simulink model "scd3busMicrogridDroopControlFidelityLevels2Inv"  (R2025b)
settings: Solver=ode15s  StartTime=0.0  StopTime=24  RelTol=1e-3
PreLoadFcn:
  | scd3busMicrogridDroopControlDataFidelityLevels2Inv;
  | 
  | %% Controller variants
  | % Create variant controls for converter controller. Controller has two
  | % different levels of fidelity: Averaged, AveragedPulse, Pulse
  | Averaged = Simulink.VariantExpression;
  | Averaged.Condition = 'fidelity==scd3busMicrogridDroopControl_variants_enum.Low';
  | Pulse = Simulink.VariantExpression;
  | Pulse.Condition = 'fidelity==scd3busMicrogridDroopControl_variants_enum.High';
  | 
  | %% Plant variants
  | % Create variant controls for converter plant. Plant has three different
  | % levels of fidelity.
  | AveragedNonSwitch = Simulink.VariantExpression;
  | AveragedNonSwitch.Condition = 'fidelity==scd3busMicrogridDroopControl_variants_enum.Low';
  | PulseSwitch = Simulink.VariantExpression;
  | PulseSwitch.Condition = 'fidelity==scd3busMicrogridDroopControl_variants_enum.High';
  | 
  | %% Set up variables ready for simulation
  | fidelity = scd3busMicrogridDroopControl_variants_enum.High;
  | Ts = 5e-6;
  | Ts_V = 1e-6;
  | Tsc = 1e-4;
  | Tsc_V = 5e-4;
values from neighbouring files (symbols this model uses):
  consensus_enable = 1    [scd3busMicrogridDroopControlDataFidelityLevels3Inv.m]
  fgrid = 60    [scd3busMicrogridDroopControlDataFidelityLevels.m]    (also in scd3busMicrogridDroopControlDataFidelityLevels3Inv.m)
  Kdroop_fp1 = 0.03/2    (= 0.015)    [scd3busMicrogridDroopControlDataFidelityLevels3Inv.m]
  Kdroop_fp2 = 0.03/2    (= 0.015)    [scd3busMicrogridDroopControlDataFidelityLevels3Inv.m]
  Kdroop_vq1 = 0.05/2    (= 0.025)    [scd3busMicrogridDroopControlDataFidelityLevels3Inv.m]
  Kdroop_vq2 = 0.05/2    (= 0.025)    [scd3busMicrogridDroopControlDataFidelityLevels3Inv.m]
  Ki_vd = 850    [scd3busMicrogridDroopControlDataFidelityLevels.m]    (also in scd3busMicrogridDroopControlDataFidelityLevels3Inv.m)
  Ki_vq = 850    [scd3busMicrogridDroopControlDataFidelityLevels.m]    (also in scd3busMicrogridDroopControlDataFidelityLevels3Inv.m)
  Kp_vd = 0.36    [scd3busMicrogridDroopControlDataFidelityLevels.m]    (also in scd3busMicrogridDroopControlDataFidelityLevels3Inv.m)
  Kp_vq = 0.36    [scd3busMicrogridDroopControlDataFidelityLevels.m]    (also in scd3busMicrogridDroopControlDataFidelityLevels3Inv.m)
  Vdc1 = 1000    [scd3busMicrogridDroopControlDataFidelityLevels.m]    (also in scd3busMicrogridDroopControlDataFidelityLevels3Inv.m)
  Vdc2 = 1000    [scd3busMicrogridDroopControlDataFidelityLevels.m]    (also in scd3busMicrogridDroopControlDataFidelityLevels3Inv.m)
  Vrms = 380    [scd3busMicrogridDroopControlDataFidelityLevels.m]    (also in scd3busMicrogridDroopControlDataFidelityLevels3Inv.m)
undefined symbols (not defined in the file or in its folder): DiscIntNeverNeededParam
libraries: ee_lib x29, nesl_utility x29, fl_lib x17, eeTransforms x4, eeSinusoidalMeasurement x4, slpidlib x4, eePwmGeneratorTwoLevel x2, eePowerMeasurement x2, simulink x2, SignalEditorBlockLib x1
(part 1 of 3)
Description:
  | Three-Phase 3 Bus Low-Inertia Microgrid Droop Control Example
settings Model: SimulationMode=rapid-accelerator  Creator=The MathWorks, Inc.  LastModifiedBy=Alex
settings SolverCC: MaxZcPerStep=1.0
settings DataIOCC: SaveOutput=off  DSMLogging=off  SaveTime=off  ReturnWorkspaceOutputs=off
settings OptimizationCC: ReuseModelBlockBuffer=off
settings DebuggingCC: StateNameClashWarn=warning
settings ModelReferenceCC: EnableRefExpFcnMdlSchedulingChecks=on
settings RTWCC: GPUComputeCapability=3.5
settings SimscapeCC: SimscapeNormalizeSystem=off

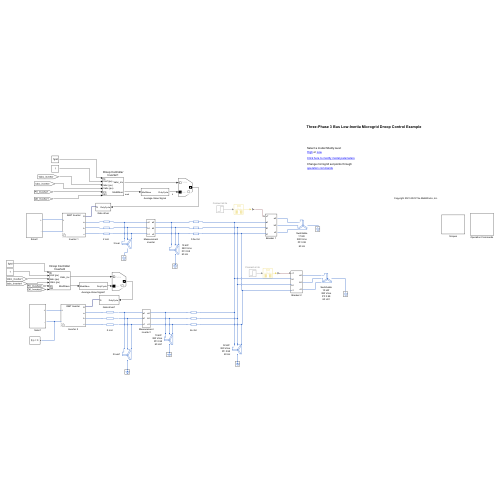
[thumbnail: Simulink's stored preview of the top-level diagram]
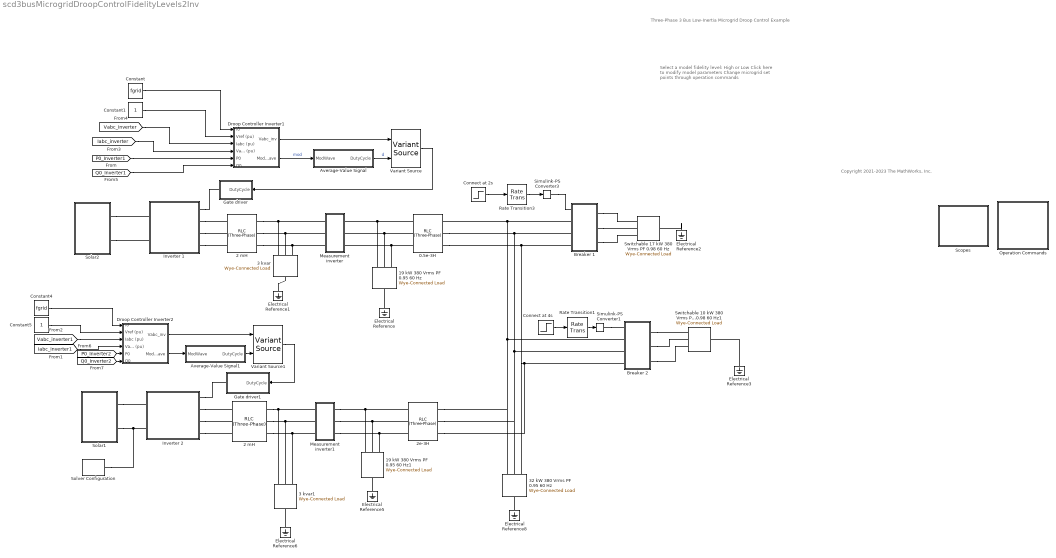
== system scd3busMicrogridDroopControlFidelityLevels2Inv ==
  note: Three-Phase 3 Bus Low-Inertia Microgrid Droop Control Example
  note: Copyright 2021-2023 The MathWorks, Inc.
  note: Select a model fidelity level:
      | High or Low
      |
      | Click here to modify model parameters
      |
      | Change microgrid set points through operation commands
  "0.5e-3H " : ee_lib/Passive/RLC Assemblies/RLC (Three-Phase)  port_option=ee.enum.threePhasePort.expanded  component_structure=ee.enum.rlc.structure.SeriesRL  R=0.02 Ohm  L=0.2e-3 H  C=1 F  R_parasitic=1e-6 Ohm  G_parasitic=1e-6 1/Ohm  IL_specify=on  IL_priority=High  IL=[0, 0, 0] A  IL_nominal_specify=off  IL_nominal_value=1  IL_nominal_unit=A  VC_specify=on  VC_priority=High  VC=[0, 0, 0] V  VC_nominal_specify=off  VC_nominal_value=1  VC_nominal_unit=V
      settings: InternalSimscapePortConfiguration="{\"Bottom\":[],\"Left\":[{\"id\":\"a1\",\"label\":\"a1\",\"type\":\"foundation.electrical.electrical\"},{\"id\":\"b1\",\"label\":\"b1\",\"type\":\"foundation.electrical.electrical\"},{\"id\":\"c1\",\"label\":\"c1\",\"type\":\"foundation.electrical.electrical\"}],\"Right\":[{\"id\":\"a2\",\"label\":\"a2\",\"type\":\"foundation.electrical.electrical\"},{\"id\":\"b2\",\"label\":\"b2\",\"type\":\"foundation.electrical.electrical\"},{\"id\":\"c2\",\"label\":\"c2\",\"type\":\"foundation.electrical.electrical\"}],\"Top\":[]}"
  19 kW 380 Vrms PF 0.95 60 Hz : ee_lib/Passive/RLC Assemblies/Wye-Connected Load  port_option=ee.enum.threePhasePort.expanded  parameterization=2  component_structure=3  component_structure_PQ=ee.enum.rlc.structure.ParallelRL  R=1 Ohm  L=0.001 H  C=1e-6 F  VRated=Vrms V  FRated=fgrid Hz  P=19000 W  Qpos=19000*sqrt(1-0.95^2)/0.95 V*A  Qneg=-3000 V*A  R_parasitic=1e-6 Ohm  G_parasitic=1e-6 1/Ohm  R_parasitic_PQ=1e-6 Ohm  G_parasitic_PQ=1e-6 1/Ohm  Vmag0=380 V  Vang0=0 deg  Freq0=60 Hz  IL_specify=on  IL_priority=High  IL=[ 0 0 0 ] A  IL_nominal_specify=off  IL_nominal_value=1  IL_nominal_unit=A  VC_specify=on  VC_priority=High  VC=[ 0 0 0 ] V  VC_nominal_specify=off  VC_nominal_value=1  VC_nominal_unit=V
      settings: InternalSimscapePortConfiguration="{\"Bottom\":[],\"Left\":[{\"id\":\"a\",\"label\":\"a\",\"type\":\"foundation.electrical.electrical\"},{\"id\":\"b\",\"label\":\"b\",\"type\":\"foundation.electrical.electrical\"},{\"id\":\"c\",\"label\":\"c\",\"type\":\"foundation.electrical.electrical\"}],\"Right\":[{\"id\":\"n\",\"label\":\"n\",\"type\":\"foundation.electrical.electrical\"}],\"Top\":[]}"
  19 kW 380 Vrms PF 0.95 60 Hz1 : ee_lib/Passive/RLC Assemblies/Wye-Connected Load  port_option=ee.enum.threePhasePort.expanded  parameterization=2  component_structure=1  component_structure_PQ=ee.enum.rlc.structure.ParallelRL  R=1 Ohm  L=0.001 H  C=1e-6 F  VRated=Vrms V  FRated=fgrid Hz  P=19000 W  Qpos=19000*sqrt(1-0.95^2)/0.95 V*A  Qneg=-3000 V*A  R_parasitic=1e-6 Ohm  G_parasitic=1e-6 1/Ohm  R_parasitic_PQ=1e-6 Ohm  G_parasitic_PQ=1e-6 1/Ohm  Vmag0=380 V  Vang0=0 deg  Freq0=60 Hz  IL_specify=on  IL_priority=High  IL=[ 0 0 0 ] A  IL_nominal_specify=off  IL_nominal_value=1  IL_nominal_unit=A  VC_specify=on  VC_priority=High  VC=[ 0 0 0 ] V  VC_nominal_specify=off  VC_nominal_value=1  VC_nominal_unit=V
      settings: InternalSimscapePortConfiguration="{\"Bottom\":[],\"Left\":[{\"id\":\"a\",\"label\":\"a\",\"type\":\"foundation.electrical.electrical\"},{\"id\":\"b\",\"label\":\"b\",\"type\":\"foundation.electrical.electrical\"},{\"id\":\"c\",\"label\":\"c\",\"type\":\"foundation.electrical.electrical\"}],\"Right\":[{\"id\":\"n\",\"label\":\"n\",\"type\":\"foundation.electrical.electrical\"}],\"Top\":[]}"
  2 mH : ee_lib/Passive/RLC Assemblies/RLC (Three-Phase)  port_option=ee.enum.threePhasePort.expanded  component_structure=ee.enum.rlc.structure.SeriesRL  R=0.02 Ohm  L=0.002 H  C=1 F  R_parasitic=1e-6 Ohm  G_parasitic=1e-6 1/Ohm  IL_specify=on  IL_priority=High  IL=[0, 0, 0] A  IL_nominal_specify=off  IL_nominal_value=1  IL_nominal_unit=A  VC_specify=on  VC_priority=High  VC=[0, 0, 0] V  VC_nominal_specify=off  VC_nominal_value=1  VC_nominal_unit=V
      settings: InternalSimscapePortConfiguration="{\"Bottom\":[],\"Left\":[{\"id\":\"a1\",\"label\":\"a1\",\"type\":\"foundation.electrical.electrical\"},{\"id\":\"b1\",\"label\":\"b1\",\"type\":\"foundation.electrical.electrical\"},{\"id\":\"c1\",\"label\":\"c1\",\"type\":\"foundation.electrical.electrical\"}],\"Right\":[{\"id\":\"a2\",\"label\":\"a2\",\"type\":\"foundation.electrical.electrical\"},{\"id\":\"b2\",\"label\":\"b2\",\"type\":\"foundation.electrical.electrical\"},{\"id\":\"c2\",\"label\":\"c2\",\"type\":\"foundation.electrical.electrical\"}],\"Top\":[]}"
  "2 mH " : ee_lib/Passive/RLC Assemblies/RLC (Three-Phase)  port_option=ee.enum.threePhasePort.expanded  component_structure=ee.enum.rlc.structure.SeriesRL  R=0.02 Ohm  L=0.002 H  C=1 F  R_parasitic=1e-6 Ohm  G_parasitic=1e-6 1/Ohm  IL_specify=on  IL_priority=High  IL=[0, 0, 0] A  IL_nominal_specify=off  IL_nominal_value=1  IL_nominal_unit=A  VC_specify=on  VC_priority=High  VC=[0, 0, 0] V  VC_nominal_specify=off  VC_nominal_value=1  VC_nominal_unit=V
      settings: InternalSimscapePortConfiguration="{\"Bottom\":[],\"Left\":[{\"id\":\"a1\",\"label\":\"a1\",\"type\":\"foundation.electrical.electrical\"},{\"id\":\"b1\",\"label\":\"b1\",\"type\":\"foundation.electrical.electrical\"},{\"id\":\"c1\",\"label\":\"c1\",\"type\":\"foundation.electrical.electrical\"}],\"Right\":[{\"id\":\"a2\",\"label\":\"a2\",\"type\":\"foundation.electrical.electrical\"},{\"id\":\"b2\",\"label\":\"b2\",\"type\":\"foundation.electrical.electrical\"},{\"id\":\"c2\",\"label\":\"c2\",\"type\":\"foundation.electrical.electrical\"}],\"Top\":[]}"
  2e-3H : ee_lib/Passive/RLC Assemblies/RLC (Three-Phase)  port_option=ee.enum.threePhasePort.expanded  component_structure=ee.enum.rlc.structure.SeriesRL  R=0.1 Ohm  L=1e-3 H  C=1 F  R_parasitic=1e-6 Ohm  G_parasitic=1e-6 1/Ohm  IL_specify=on  IL_priority=High  IL=[0, 0, 0] A  IL_nominal_specify=off  IL_nominal_value=1  IL_nominal_unit=A  VC_specify=on  VC_priority=High  VC=[0, 0, 0] V  VC_nominal_specify=off  VC_nominal_value=1  VC_nominal_unit=V
      settings: InternalSimscapePortConfiguration="{\"Bottom\":[],\"Left\":[{\"id\":\"a1\",\"label\":\"a1\",\"type\":\"foundation.electrical.electrical\"},{\"id\":\"b1\",\"label\":\"b1\",\"type\":\"foundation.electrical.electrical\"},{\"id\":\"c1\",\"label\":\"c1\",\"type\":\"foundation.electrical.electrical\"}],\"Right\":[{\"id\":\"a2\",\"label\":\"a2\",\"type\":\"foundation.electrical.electrical\"},{\"id\":\"b2\",\"label\":\"b2\",\"type\":\"foundation.electrical.electrical\"},{\"id\":\"c2\",\"label\":\"c2\",\"type\":\"foundation.electrical.electrical\"}],\"Top\":[]}"
  3 kvar : ee_lib/Passive/RLC Assemblies/Wye-Connected Load  port_option=ee.enum.threePhasePort.expanded  parameterization=2  component_structure=3  component_structure_PQ=3  R=1 Ohm  L=0.001 H  C=1e-6 F  VRated=Vrms V  FRated=fgrid Hz  P=0 W  Qpos=0 V*A  Qneg=-3000 V*A  R_parasitic=1e-6 Ohm  G_parasitic=1e-6 1/Ohm  R_parasitic_PQ=1e-6 Ohm  G_parasitic_PQ=1e-6 1/Ohm  Vmag0=380 V  Vang0=0 deg  Freq0=60 Hz  IL_specify=on  IL_priority=High  IL=[ 0 0 0 ] A  IL_nominal_specify=off  IL_nominal_value=1  IL_nominal_unit=A  VC_specify=on  VC_priority=High  VC=[ 0 0 0 ] V  VC_nominal_specify=off  VC_nominal_value=1  VC_nominal_unit=V
      settings: InternalSimscapePortConfiguration="{\"Bottom\":[],\"Left\":[{\"id\":\"a\",\"label\":\"a\",\"type\":\"foundation.electrical.electrical\"},{\"id\":\"b\",\"label\":\"b\",\"type\":\"foundation.electrical.electrical\"},{\"id\":\"c\",\"label\":\"c\",\"type\":\"foundation.electrical.electrical\"}],\"Right\":[{\"id\":\"n\",\"label\":\"n\",\"type\":\"foundation.electrical.electrical\"}],\"Top\":[]}"
  3 kvar1 : ee_lib/Passive/RLC Assemblies/Wye-Connected Load  port_option=ee.enum.threePhasePort.expanded  parameterization=ee.enum.rlc.parameterization.ratedpower  component_structure=ee.enum.rlc.structure.C  component_structure_PQ=ee.enum.rlc.structure.C  R=1 Ohm  L=0.001 H  C=1e-6 F  VRated=Vrms V  FRated=fgrid Hz  P=0 W  Qpos=0 A*V  Qneg=-3000 A*V  R_parasitic=1e-6 Ohm  G_parasitic=1e-6 1/Ohm  R_parasitic_PQ=1e-6 Ohm  G_parasitic_PQ=1e-6 1/Ohm  Vmag0=380 V  Vang0=0 deg  Freq0=60 Hz  IL_specify=on  IL_priority=High  IL=[ 0 0 0 ] A  IL_nominal_specify=off  IL_nominal_value=1  IL_nominal_unit=A  VC_specify=on  VC_priority=High  VC=[ 0 0 0 ] V  VC_nominal_specify=off  VC_nominal_value=1  VC_nominal_unit=V
      settings: InternalSimscapePortConfiguration="{\"Bottom\":[],\"Left\":[{\"id\":\"a\",\"label\":\"a\",\"type\":\"foundation.electrical.electrical\"},{\"id\":\"b\",\"label\":\"b\",\"type\":\"foundation.electrical.electrical\"},{\"id\":\"c\",\"label\":\"c\",\"type\":\"foundation.electrical.electrical\"}],\"Right\":[{\"id\":\"n\",\"label\":\"n\",\"type\":\"foundation.electrical.electrical\"}],\"Top\":[]}"
  32 kW 380 Vrms PF 0.95 60 Hz : ee_lib/Passive/RLC Assemblies/Wye-Connected Load  port_option=ee.enum.threePhasePort.expanded  parameterization=2  component_structure=3  component_structure_PQ=ee.enum.rlc.structure.ParallelRL  R=1 Ohm  L=0.001 H  C=1e-6 F  VRated=Vrms V  FRated=fgrid Hz  P=32000 W  Qpos=32000*sqrt(1-0.95^2)/0.95 V*A  Qneg=-3000 V*A  R_parasitic=1e-6 Ohm  G_parasitic=1e-6 1/Ohm  R_parasitic_PQ=1e-6 Ohm  G_parasitic_PQ=1e-6 1/Ohm  Vmag0=380 V  Vang0=0 deg  Freq0=60 Hz  IL_specify=on  IL_priority=High  IL=[ 0 0 0 ] A  IL_nominal_specify=off  IL_nominal_value=1  IL_nominal_unit=A  VC_specify=on  VC_priority=High  VC=[ 0 0 0 ] V  VC_nominal_specify=off  VC_nominal_value=1  VC_nominal_unit=V
      settings: InternalSimscapePortConfiguration="{\"Bottom\":[],\"Left\":[{\"id\":\"a\",\"label\":\"a\",\"type\":\"foundation.electrical.electrical\"},{\"id\":\"b\",\"label\":\"b\",\"type\":\"foundation.electrical.electrical\"},{\"id\":\"c\",\"label\":\"c\",\"type\":\"foundation.electrical.electrical\"}],\"Right\":[{\"id\":\"n\",\"label\":\"n\",\"type\":\"foundation.electrical.electrical\"}],\"Top\":[]}"
  Average-Value Signal : Subsystem
  Average-Value Signal1 : Subsystem
  Breaker 1 : Subsystem
  Breaker 2 : Subsystem
  Connect at 2s : Step  Time=6  SampleTime=0
  Connect at 4s : Step  Time=10  SampleTime=0
  Constant : Constant  Value=fgrid
  Constant1 : Constant
  Constant4 : Constant  Value=fgrid
  Constant5 : Constant
  Droop Controller Inverter1 : Subsystem
  Droop Controller Inverter2 : Subsystem
  Electrical Reference{,1..3,5..6,8} (7 alike) : fl_lib/Electrical/Electrical Elements/Electrical Reference
  Gate driver : Subsystem
  Gate driver1 : Subsystem
  Inverter 1 : Subsystem  Variant=on  VariantControl=Choice
  Inverter 2 : Subsystem  Variant=on  VariantControl=Choice
  Measurement inverter : Subsystem
  Measurement inverter1 : Subsystem
  Operation Commands : Subsystem
  Rate Transition1 : RateTransition  Integrity=off  OutPortSampleTimeOpt=Inherit
  Rate Transition3 : RateTransition  Integrity=off  OutPortSampleTimeOpt=Inherit
  Scopes : Subsystem
  Simulink-PS Converter1 : nesl_utility/Simulink-PS Converter  PhysicalDomain=network_engine_domain  SubClassName=ps_input  LeftPortType=input  RightPortType=output  PseudoPeriodic=off  Frequencies=[]  NoiseDistribution=none  NoiseParameters=[]  Unit=1  AffineConversion=off  FilteringAndDerivatives=provide  SimscapeFilterOrder=1  InputFilterTimeConstant=0.001  UdotUserProvided=0
  Simulink-PS Converter3 : nesl_utility/Simulink-PS Converter  PhysicalDomain=network_engine_domain  SubClassName=ps_input  LeftPortType=input  RightPortType=output  PseudoPeriodic=off  Frequencies=[]  NoiseDistribution=none  NoiseParameters=[]  Unit=1  AffineConversion=off  FilteringAndDerivatives=provide  SimscapeFilterOrder=1  InputFilterTimeConstant=0.001  UdotUserProvided=0
  Solar1 : Subsystem
  Solar2 : Subsystem
  Solver Configuration : nesl_utility/Solver Configuration  PhysicalDomain=network_engine_domain  SubClassName=solver  LeftPortType=input  RightPortType=generic  Tones=[]  Harmonics=[]  SimulateNoise=off  Profile=off  UseLocalSampling=off  EnableSwitchedLinearOptims=on  FrequencyDomain=off  UseCCode=off  RelTol=0.001  AbsTol=1e-06  MinStep=1e-09  ToWorkspace=off  RevertToSquareIcSolve=off  NumHomotopyIterations=100  PhasorMode=off  PhasorModeNumHarmonics=1  ConsistencySolver=NEWTON_FTOL  IndexReductionMethod=DerivativeReplacement  DoDC=off  ResidualTolerance=1e-09  ConsistencyTolSource=GLOBAL  ConsistencyAbsTol=0.001  ConsistencyRelTol=0.001  ConsistencyTolFactor=0.001  UseLocalSolver=on  LocalSolverChoice=NE_BACKWARD_EULER_ADVANCER  ResolveIndetEquations=on  FunctionEvalNumThread=1  LocalSolverSampleTime=Ts  DoFixedCost=off  MaxNonlinIter=3  MaxModeIter=2  ComputeImpulses=off  ImpulseIterations=1  LinearAlgebra=auto  LinearAlgebraNumThread=0  EquationFormulation=NE_TIME_EF  DelaysMemoryBudget=1024  AutomaticFiltering=on  FilteringTimeConstant=0.001  PartitionStorageMethod=AS_NEEDED  PartitionMemoryBudget=1024  PartitionMethod=FAST  MultibodyUseLocalSolver=off  MultibodyLocalSolverChoice=ODE1  MultibodyLocalSolverSampleTime=0.001
  Switchable 10 kW 380 Vrms PF 0.98 60 Hz1 : ee_lib/Passive/RLC Assemblies/Wye-Connected Load  port_option=ee.enum.threePhasePort.expanded  parameterization=2  component_structure=3  component_structure_PQ=ee.enum.rlc.structure.ParallelRL  R=1 Ohm  L=0.001 H  C=1e-6 F  VRated=Vrms V  FRated=fgrid Hz  P=10000 W  Qpos=10000*sqrt(1-0.98^2)/0.98 V*A  Qneg=-3000 V*A  R_parasitic=1e-6 Ohm  G_parasitic=1e-6 1/Ohm  R_parasitic_PQ=1e-6 Ohm  G_parasitic_PQ=1e-6 1/Ohm  Vmag0=380 V  Vang0=0 deg  Freq0=60 Hz  IL_specify=on  IL_priority=High  IL=[ 0 0 0 ] A  IL_nominal_specify=off  IL_nominal_value=1  IL_nominal_unit=A  VC_specify=on  VC_priority=High  VC=[ 0 0 0 ] V  VC_nominal_specify=off  VC_nominal_value=1  VC_nominal_unit=V
      settings: InternalSimscapePortConfiguration="{\"Bottom\":[],\"Left\":[{\"id\":\"a\",\"label\":\"a\",\"type\":\"foundation.electrical.electrical\"},{\"id\":\"b\",\"label\":\"b\",\"type\":\"foundation.electrical.electrical\"},{\"id\":\"c\",\"label\":\"c\",\"type\":\"foundation.electrical.electrical\"}],\"Right\":[{\"id\":\"n\",\"label\":\"n\",\"type\":\"foundation.electrical.electrical\"}],\"Top\":[]}"
  Switchable 17 kW 380 Vrms PF 0.98 60 Hz : ee_lib/Passive/RLC Assemblies/Wye-Connected Load  port_option=ee.enum.threePhasePort.expanded  parameterization=2  component_structure=3  component_structure_PQ=ee.enum.rlc.structure.ParallelRL  R=1 Ohm  L=0.001 H  C=1e-6 F  VRated=Vrms V  FRated=fgrid Hz  P=17000 W  Qpos=17000*sqrt(1-0.98^2)/0.98 V*A  Qneg=-3000 V*A  R_parasitic=1e-6 Ohm  G_parasitic=1e-6 1/Ohm  R_parasitic_PQ=1e-6 Ohm  G_parasitic_PQ=1e-6 1/Ohm  Vmag0=380 V  Vang0=0 deg  Freq0=60 Hz  IL_specify=on  IL_priority=High  IL=[ 0 0 0 ] A  IL_nominal_specify=off  IL_nominal_value=1  IL_nominal_unit=A  VC_specify=on  VC_priority=High  VC=[ 0 0 0 ] V  VC_nominal_specify=off  VC_nominal_value=1  VC_nominal_unit=V
      settings: InternalSimscapePortConfiguration="{\"Bottom\":[],\"Left\":[{\"id\":\"a\",\"label\":\"a\",\"type\":\"foundation.electrical.electrical\"},{\"id\":\"b\",\"label\":\"b\",\"type\":\"foundation.electrical.electrical\"},{\"id\":\"c\",\"label\":\"c\",\"type\":\"foundation.electrical.electrical\"}],\"Right\":[{\"id\":\"n\",\"label\":\"n\",\"type\":\"foundation.electrical.electrical\"}],\"Top\":[]}"
  Variant Source : VariantSource  ShowConditionOnBlock=on  VariantControls={Pulse, Averaged}
  Variant Source1 : VariantSource  ShowConditionOnBlock=on  VariantControls={Pulse, Averaged}
  wires:
  [Vabc_inverter] -> Droop Controller Inverter1/3(Iabc (pu))
  Constant1/1 -> Droop Controller Inverter1/2(Vref (pu))
  [Iabc_inverter] -> Droop Controller Inverter1/4(Vabc (pu))
  [P0_Inverter1] -> Droop Controller Inverter1/5(P0)
  Variant Source/1 -> Gate driver/1(DutyCycle)
  Average-Value Signal/1(DutyCycle) -> Variant Source/2  "d"
  Droop Controller Inverter1/1(Vabc_inv) -> Variant Source/1
  Constant/1 -> Droop Controller Inverter1/1(f0)
  [Q0_Inverter1] -> Droop Controller Inverter1/6(Q0)
  Rate Transition3/1 -> Simulink-PS Converter3/1
  Droop Controller Inverter1/2(ModWave) -> Average-Value Signal/1(ModWave)  "mod"
  Connect at 2s/1 -> Rate Transition3/1
  Connect at 4s/1 -> Rate Transition1/1
  Rate Transition1/1 -> Simulink-PS Converter1/1
  Droop Controller Inverter2/2(ModWave) -> Average-Value Signal1/1(ModWave)
  [Q0_Inverter2] -> Droop Controller Inverter2/6(Q0)
  [P0_Inverter2] -> Droop Controller Inverter2/5(P0)
  Constant4/1 -> Droop Controller Inverter2/1(f0)
  Constant5/1 -> Droop Controller Inverter2/2(Vref (pu))
  [Iabc_inverter1] -> Droop Controller Inverter2/4(Vabc (pu))
  [Vabc_inverter1] -> Droop Controller Inverter2/3(Iabc (pu))
  Average-Value Signal1/1(DutyCycle) -> Variant Source1/2
  Droop Controller Inverter2/1(Vabc_inv) -> Variant Source1/1
  Variant Source1/1 -> Gate driver1/1(DutyCycle)
  connections:
  Measurement inverter/LConn1 -- "2 mH "/RConn1 -- 3 kvar/LConn1
  Breaker 1/LConn4 -- "0.5e-3H "/RConn3 -- Breaker 2/LConn4 -- 2e-3H/RConn3 -- 32 kW 380 Vrms PF 0.95 60 Hz/LConn3
  Measurement inverter/LConn3 -- "2 mH "/RConn3 -- 3 kvar/LConn3
  Measurement inverter/LConn2 -- "2 mH "/RConn2 -- 3 kvar/LConn2
  Electrical Reference1/LConn1 -- 3 kvar/RConn1
  Electrical Reference2/LConn1 -- Switchable 17 kW 380 Vrms PF 0.98 60 Hz/RConn1
  Breaker 1/RConn2 -- Switchable 17 kW 380 Vrms PF 0.98 60 Hz/LConn2
  Electrical Reference/LConn1 -- 19 kW 380 Vrms PF 0.95 60 Hz/RConn1
  Electrical Reference8/LConn1 -- 32 kW 380 Vrms PF 0.95 60 Hz/RConn1
  Inverter 1/LConn1 -- Gate driver/RConn1
  Inverter 1/LConn2 -- "2 mH "/LConn1
  Simulink-PS Converter3/RConn1 -- Breaker 1/LConn1
  Inverter 1/LConn4 -- "2 mH "/LConn3
  Inverter 1/LConn3 -- "2 mH "/LConn2
  Breaker 1/RConn3 -- Switchable 17 kW 380 Vrms PF 0.98 60 Hz/LConn3
  Breaker 1/RConn1 -- Switchable 17 kW 380 Vrms PF 0.98 60 Hz/LConn1
  Solar2/RConn2 -- Inverter 1/RConn2
  Solar2/RConn1 -- Inverter 1/RConn1
  Breaker 2/RConn2 -- Switchable 10 kW 380 Vrms PF 0.98 60 Hz1/LConn2
  Electrical Reference3/LConn1 -- Switchable 10 kW 380 Vrms PF 0.98 60 Hz1/RConn1
  Breaker 2/RConn3 -- Switchable 10 kW 380 Vrms PF 0.98 60 Hz1/LConn3
  Breaker 2/RConn1 -- Switchable 10 kW 380 Vrms PF 0.98 60 Hz1/LConn1
  Simulink-PS Converter1/RConn1 -- Breaker 2/LConn1
  19 kW 380 Vrms PF 0.95 60 Hz/LConn1 -- "0.5e-3H "/LConn1 -- Measurement inverter/RConn1
  19 kW 380 Vrms PF 0.95 60 Hz/LConn2 -- "0.5e-3H "/LConn2 -- Measurement inverter/RConn2
  19 kW 380 Vrms PF 0.95 60 Hz/LConn3 -- "0.5e-3H "/LConn3 -- Measurement inverter/RConn3
  Breaker 2/LConn2 -- 2e-3H/RConn1 -- 32 kW 380 Vrms PF 0.95 60 Hz/LConn1 -- Breaker 1/LConn2 -- "0.5e-3H "/RConn1
  Breaker 1/LConn3 -- "0.5e-3H "/RConn2 -- 2e-3H/RConn2 -- 32 kW 380 Vrms PF 0.95 60 Hz/LConn2 -- Breaker 2/LConn3
  Inverter 2/LConn3 -- 2 mH/LConn2
  Inverter 2/LConn4 -- 2 mH/LConn3
  Measurement inverter1/RConn1 -- 2e-3H/LConn1 -- 19 kW 380 Vrms PF 0.95 60 Hz1/LConn1
  Inverter 2/LConn2 -- 2 mH/LConn1
  Electrical Reference5/LConn1 -- 19 kW 380 Vrms PF 0.95 60 Hz1/RConn1
  2 mH/RConn1 -- Measurement inverter1/LConn1 -- 3 kvar1/LConn1
  Measurement inverter1/RConn2 -- 2e-3H/LConn2 -- 19 kW 380 Vrms PF 0.95 60 Hz1/LConn2
  Solar1/RConn1 -- Inverter 2/RConn1
  2 mH/RConn3 -- Measurement inverter1/LConn3 -- 3 kvar1/LConn3
  2e-3H/LConn3 -- Measurement inverter1/RConn3 -- 19 kW 380 Vrms PF 0.95 60 Hz1/LConn3
  Inverter 2/LConn1 -- Gate driver1/RConn1
  2 mH/RConn2 -- Measurement inverter1/LConn2 -- 3 kvar1/LConn2
  Electrical Reference6/LConn1 -- 3 kvar1/RConn1
  Solar1/RConn2 -- Solver Configuration/RConn1 -- Inverter 2/RConn2

== system scd3busMicrogridDroopControlFidelityLevels2Inv/Average-Value Signal ==
  ModWave : Inport
  Bias : Bias  Bias=1  SaturateOnIntegerOverflow=off
  Bias1 : Bias  Bias=1  SaturateOnIntegerOverflow=off
  Gain : Gain  Gain=-1
  Mod. Index1 : Gain  Gain=0.5
  Mux : Mux  Inputs=2
  Rate Transition : RateTransition  OutPortSampleTime=Ts_V
  Selector4 : Selector  InputPortWidth=6  IndexOptions=Index vector (dialog)  Indices=[1 4 2 5 3 6]  OutputSizes=1
  DutyCycle : Outport
  wires:
  Mux/1 -> Selector4/1
  Bias1/1 -> Mux/2
  Selector4/1 -> DutyCycle/1
  Rate Transition/1 -> Bias/1
  Bias/1 -> Mod. Index1/1
  Mod. Index1/1 -> Mux/1, Gain/1
  Gain/1 -> Bias1/1
  ModWave/1 -> Rate Transition/1

== system scd3busMicrogridDroopControlFidelityLevels2Inv/Average-Value Signal1 ==
  ModWave : Inport
  Bias : Bias  Bias=1  SaturateOnIntegerOverflow=off
  Bias1 : Bias  Bias=1  SaturateOnIntegerOverflow=off
  Gain : Gain  Gain=-1
  Mod. Index1 : Gain  Gain=0.5
  Mux : Mux  Inputs=2
  Rate Transition : RateTransition  OutPortSampleTime=Ts_V
  Selector4 : Selector  InputPortWidth=6  IndexOptions=Index vector (dialog)  Indices=[1 4 2 5 3 6]  OutputSizes=1
  DutyCycle : Outport
  wires:
  ModWave/1 -> Rate Transition/1
  Gain/1 -> Bias1/1
  Mod. Index1/1 -> Gain/1, Mux/1
  Bias/1 -> Mod. Index1/1
  Rate Transition/1 -> Bias/1
  Selector4/1 -> DutyCycle/1
  Bias1/1 -> Mux/2
  Mux/1 -> Selector4/1

== system scd3busMicrogridDroopControlFidelityLevels2Inv/Breaker 1 ==
  SPST Switch : ee_lib/Switches & Breakers/SPST Switch  R_closed=0.01 Ohm  G_open=1e-6 S  Threshold=0.5 V  Width=0 V  model_dynamics=0  t_on=1e-3 s  t_off=1e-3 s  initial_vT=0 V
      settings: InternalSimscapePortConfiguration="{\"Bottom\":[],\"Left\":[{\"id\":\"vT\",\"label\":\"vT\",\"type\":\"input\"},{\"id\":\"p\",\"label\":\"\",\"type\":\"foundation.electrical.electrical\"}],\"Right\":[{\"id\":\"n\",\"label\":\"\",\"type\":\"foundation.electrical.electrical\"}],\"Top\":[]}"
  SPST Switch1 : ee_lib/Switches & Breakers/SPST Switch  R_closed=0.01 Ohm  G_open=1e-6 S  Threshold=0.5 V  Width=0 V  model_dynamics=0  t_on=1e-3 s  t_off=1e-3 s  initial_vT=0 V
      settings: InternalSimscapePortConfiguration="{\"Bottom\":[],\"Left\":[{\"id\":\"vT\",\"label\":\"vT\",\"type\":\"input\"},{\"id\":\"p\",\"label\":\"\",\"type\":\"foundation.electrical.electrical\"}],\"Right\":[{\"id\":\"n\",\"label\":\"\",\"type\":\"foundation.electrical.electrical\"}],\"Top\":[]}"
  SPST Switch2 : ee_lib/Switches & Breakers/SPST Switch  R_closed=0.01 Ohm  G_open=1e-6 S  Threshold=0.5 V  Width=0 V  model_dynamics=0  t_on=1e-3 s  t_off=1e-3 s  initial_vT=0 V
      settings: InternalSimscapePortConfiguration="{\"Bottom\":[],\"Left\":[{\"id\":\"vT\",\"label\":\"vT\",\"type\":\"input\"},{\"id\":\"p\",\"label\":\"\",\"type\":\"foundation.electrical.electrical\"}],\"Right\":[{\"id\":\"n\",\"label\":\"\",\"type\":\"foundation.electrical.electrical\"}],\"Top\":[]}"
  vT : PMIOPort  Side=Left
  a1 : PMIOPort  Port=2  Side=Left
  b1 : PMIOPort  Port=3  Side=Left
  c1 : PMIOPort  Port=4  Side=Left
  a2 : PMIOPort  Port=5  Side=Right
  b2 : PMIOPort  Port=6  Side=Right
  c2 : PMIOPort  Port=7  Side=Right
  connections:
  SPST Switch1/RConn1 -- b2/RConn1
  SPST Switch2/RConn1 -- a2/RConn1
  SPST Switch/LConn1 -- SPST Switch1/LConn1 -- vT/RConn1 -- SPST Switch2/LConn1
  SPST Switch/RConn1 -- c2/RConn1
  SPST Switch2/LConn2 -- a1/RConn1
  SPST Switch/LConn2 -- c1/RConn1
  SPST Switch1/LConn2 -- b1/RConn1

== system scd3busMicrogridDroopControlFidelityLevels2Inv/Breaker 2 ==
  SPST Switch : ee_lib/Switches & Breakers/SPST Switch  R_closed=0.01 Ohm  G_open=1e-6 S  Threshold=0.5 V  Width=0 V  model_dynamics=0  t_on=1e-3 s  t_off=1e-3 s  initial_vT=0 V
      settings: InternalSimscapePortConfiguration="{\"Bottom\":[],\"Left\":[{\"id\":\"vT\",\"label\":\"vT\",\"type\":\"input\"},{\"id\":\"p\",\"label\":\"\",\"type\":\"foundation.electrical.electrical\"}],\"Right\":[{\"id\":\"n\",\"label\":\"\",\"type\":\"foundation.electrical.electrical\"}],\"Top\":[]}"
  SPST Switch1 : ee_lib/Switches & Breakers/SPST Switch  R_closed=0.01 Ohm  G_open=1e-6 S  Threshold=0.5 V  Width=0 V  model_dynamics=0  t_on=1e-3 s  t_off=1e-3 s  initial_vT=0 V
      settings: InternalSimscapePortConfiguration="{\"Bottom\":[],\"Left\":[{\"id\":\"vT\",\"label\":\"vT\",\"type\":\"input\"},{\"id\":\"p\",\"label\":\"\",\"type\":\"foundation.electrical.electrical\"}],\"Right\":[{\"id\":\"n\",\"label\":\"\",\"type\":\"foundation.electrical.electrical\"}],\"Top\":[]}"
  SPST Switch2 : ee_lib/Switches & Breakers/SPST Switch  R_closed=0.01 Ohm  G_open=1e-6 S  Threshold=0.5 V  Width=0 V  model_dynamics=0  t_on=1e-3 s  t_off=1e-3 s  initial_vT=0 V
      settings: InternalSimscapePortConfiguration="{\"Bottom\":[],\"Left\":[{\"id\":\"vT\",\"label\":\"vT\",\"type\":\"input\"},{\"id\":\"p\",\"label\":\"\",\"type\":\"foundation.electrical.electrical\"}],\"Right\":[{\"id\":\"n\",\"label\":\"\",\"type\":\"foundation.electrical.electrical\"}],\"Top\":[]}"
  vT : PMIOPort  Side=Left
  a1 : PMIOPort  Port=2  Side=Left
  b1 : PMIOPort  Port=3  Side=Left
  c1 : PMIOPort  Port=4  Side=Left
  a2 : PMIOPort  Port=5  Side=Right
  b2 : PMIOPort  Port=6  Side=Right
  c2 : PMIOPort  Port=7  Side=Right
  connections:
  SPST Switch1/RConn1 -- b2/RConn1
  SPST Switch2/RConn1 -- a2/RConn1
  SPST Switch/LConn1 -- SPST Switch1/LConn1 -- vT/RConn1 -- SPST Switch2/LConn1
  SPST Switch/RConn1 -- c2/RConn1
  SPST Switch2/LConn2 -- a1/RConn1
  SPST Switch/LConn2 -- c1/RConn1
  SPST Switch1/LConn2 -- b1/RConn1

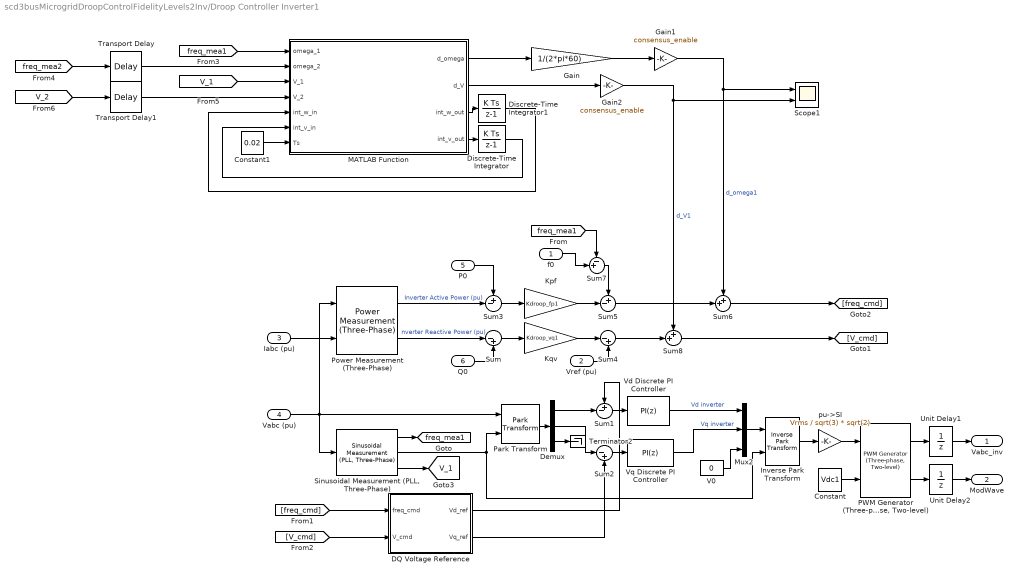
== system scd3busMicrogridDroopControlFidelityLevels2Inv/Droop Controller Inverter1 ==
  f0 : Inport
  Vref (pu) : Inport  Port=2
  Iabc (pu) : Inport  Port=3
  Vabc (pu) : Inport  Port=4
  P0 : Inport  Port=5
  Q0 : Inport  Port=6
  Constant : Constant  Value=Vdc1
  Constant1 : Constant  Value=0.02
  DQ Voltage Reference : Subsystem
  Demux : Demux  Outputs=3
  Discrete-Time Integrator : DiscreteIntegrator  SampleTime=0.02  ICPrevOutput=DiscIntNeverNeededParam  ICPrevScaledInput=DiscIntNeverNeededParam
  Discrete-Time Integrator1 : DiscreteIntegrator  SampleTime=0.02  ICPrevOutput=DiscIntNeverNeededParam  ICPrevScaledInput=DiscIntNeverNeededParam
  Gain : Gain  Gain=1/(2*pi*60)
  Gain1 : Gain  Gain=consensus_enable
  Gain2 : Gain  Gain=consensus_enable
  Inverse Park Transform : eeTransforms/Inverse Park Transform  AxisAlignment=Q-axis  PowerInvariant=off
  Kpf : Gain  Gain=Kdroop_fp1
  Kqv : Gain  Gain=Kdroop_vq1
  MATLAB Function : MATLAB Function  TreatAsAtomicUnit=on
  Mux2 : Mux  Inputs=3
  "PWM Generator (Three-phase, Two-level)" : eePwmGeneratorTwoLevel/PWM Generator (Three-phase, Two-level)  PWMMode=Continuous PWM (CPWM)  CPWMMode=SPWM: sinusoidal PWM  DPWMMode=60 DPWM: 60 degree discontinuous PWM  fsw=fsw_V  Ts=Ts_V
  Park Transform : eeTransforms/Park Transform  AxisAlignment=Q-axis  PowerInvariant=off
  Power Measurement (Three-Phase) : eePowerMeasurement/Power Measurement (Three-Phase)  LabelModeActiveChoice=Discrete  F=fgrid  K=1  Seq=Positive  Ts=Ts
  Scope1 : Scope  NumInputPorts=2
      settings: ActiveDisplayYMinimum=-0.0066314559621623061  ActiveDisplayYMaximum=0.0066314559621623061  DataLoggingVariableName=ScopeData3
  "Sinusoidal Measurement (PLL, Three-Phase)" : eeSinusoidalMeasurement/Sinusoidal Measurement (PLL, Three-Phase)  Kp_LF=180  Ki_LF=3200  F0=fgrid  Theta0=0  Ts=Ts_V
  Sum : Sum  Inputs=|-+
  Sum1 : Sum  Inputs=+-|  InputSameDT=on  SaturateOnIntegerOverflow=on  OutDataTypeStr=Inherit: Same as first input
  Sum2 : Sum  Inputs=|-+  InputSameDT=on  SaturateOnIntegerOverflow=on  OutDataTypeStr=Inherit: Same as first input
  Sum3 : Sum  Inputs=+-|
  Sum4 : Sum  Inputs=|-+
  Sum5 : Sum  Inputs=+-|
  Sum6 : Sum  Inputs=++|
  Sum7 : Sum  Inputs=-+|
  Sum8 : Sum  Inputs=++|
  Terminator2 : Terminator
  Transport Delay : TransportDelay  DelayTime=0.1
  Transport Delay1 : TransportDelay  DelayTime=0.1
  Unit Delay1 : UnitDelay  SampleTime=Ts_V  HasFrameUpgradeWarning=on
  Unit Delay2 : UnitDelay  SampleTime=Ts_V  HasFrameUpgradeWarning=on
  V0 : Constant  Value=0
  Vd Discrete PI Controller : slpidlib/PID Controller  Controller=PI  Form=Parallel  TimeDomain=Discrete-time  UseExternalTs=off  SampleTime=Ts_V  IntegratorMethod=Forward Euler  FilterMethod=Forward Euler  ControllerParametersSource=internal  P=Kp_vd  I=Ki_vd  UseKiTs=off  D=0  UseExternalDerivativeSource=off  N=100  UseFilter=on  TunerSelectOption=Transfer Function Based (PID Tuner App)  InitialConditionSource=internal  InitialConditionForIntegrator=0.62  InitialConditionForFilter=0  DifferentiatorICPrevScaledInput=0  ExternalReset=none  TrackingMode=off  Kt=1  LimitOutput=on  SatLimitsSource=internal  UpperSaturationLimit=1  LowerSaturationLimit=0  LinearizeAsGain=on  AntiWindupMode=none  Kb=1  LimitIntegrator=off  UpperIntegratorSaturationLimit=inf  LowerIntegratorSaturationLimit=-inf  POutMin=[]  POutMax=[]  IOutMin=[]  IOutMax=[]  DOutMin=[]  DOutMax=[]  NOutMin=[]  NOutMax=[]  SumOutMin=[]  SumOutMax=[]  SaturationOutMin=[]  SaturationOutMax=[]  PParamMin=[]  PParamMax=[]  IParamMin=[]  IParamMax=[]  DParamMin=[]  DParamMax=[]  NParamMin=[]  NParamMax=[]  KbParamMin=[]  KbParamMax=[]  KtParamMin=[]  KtParamMax=[]  KbOutMin=[]  KbOutMax=[]  KtOutMin=[]  KtOutMax=[]  IntegratorOutMin=[]  IntegratorOutMax=[]  FilterOutMin=[]  FilterOutMax=[]  SumI1OutMin=[]  SumI1OutMax=[]  SumI2OutMin=[]  SumI2OutMax=[]  SumI3OutMin=[]  SumI3OutMax=[]  SumI4OutMin=[]  SumI4OutMax=[]  SumDOutMin=[]  SumDOutMax=[]  DifferentiatorOutMin=[]  DifferentiatorOutMax=[]  FilterDiffOutCoefMin=[]  FilterDiffOutCoefMax=[]  ReciprocalOutMin=[]  ReciprocalOutMax=[]  SumDenOutMin=[]  SumDenOutMax=[]  SumNumOutMin=[]  SumNumOutMax=[]  DivideOutMin=[]  DivideOutMax=[]  UdiffTsProdOutMin=[]  UdiffTsProdOutMax=[]  NTsProdOutMin=[]  NTsProdOutMax=[]  UintegralTsProdOutMin=[]  UintegralTsProdOutMax=[]  UngainTsProdOutMin=[]  UngainTsProdOutMax=[]  ClampingZeroOutDataTypeStr=Inherit: Inherit via back propagation  ClampingZeroOutMin=[]  ClampingZeroOutMax=[]  FilterDenConstantOutDataTypeStr=Inherit: Inherit via back propagation  FilterDenConstantOutMin=[]  FilterDenConstantOutMax=[]  PCopyOutDataTypeStr=Inherit: Inherit via back propagation  PCopyOutMin=[]  PCopyOutMax=[]  NCopyOutDataTypeStr=Inherit: Inherit via back propagation  NCopyOutMin=[]  NCopyOutMax=[]  IntegratorContinuousStateAttributes=''  IntegratorStateMustResolveToSignalObject=off  IntegratorRTWStateStorageClass=Auto  FilterContinuousStateAttributes=''  FilterStateMustResolveToSignalObject=off  FilterRTWStateStorageClass=Auto  ParallelPVariant=InternalParameters  IdealPVariant=Disabled  IVariant=InternalParameters  DVariant=Disabled  IntegratorVariant=Discrete  SatVariant=Enabled  AWVariant=Passthrough  PCopyVariant=Disabled  TRVariant=Disabled  FdbkBlocksVariant=Forward  IdealPFdbkVariant=Disabled  SatFdbkVariant=Disabled  DerivativeFilterVariant=Disabled  NVariant=Disabled  NCopyVariant=Disabled_SignalSpec  FilterICVariant=Disabled  IntegratorICVariant=InternalICs  ExternalResetVariant=Disabled  TRSumVariant=Passthrough  SumFdbkVariant=Disabled  SumVariant=Sum_PI  TsampFilterVariant=InternalTs  TsampNgainVariant=Passthrough  TsampIntegralVariant=Disabled_SignalSpec  ExternalSaturationOutDataTypeStr=Inherit: Same as second input  DerivativeSourceVariant=Disabled  PreIntVariant=InternalPreInt
  Vq Discrete PI Controller : slpidlib/PID Controller  Controller=PI  Form=Parallel  TimeDomain=Discrete-time  UseExternalTs=off  SampleTime=Ts_V  IntegratorMethod=Forward Euler  FilterMethod=Forward Euler  ControllerParametersSource=internal  P=Kp_vq  I=Ki_vq  UseKiTs=off  D=0  UseExternalDerivativeSource=off  N=100  UseFilter=on  TunerSelectOption=Transfer Function Based (PID Tuner App)  InitialConditionSource=internal  InitialConditionForIntegrator=0  InitialConditionForFilter=0  DifferentiatorICPrevScaledInput=0  ExternalReset=none  TrackingMode=off  Kt=1  LimitOutput=on  SatLimitsSource=internal  UpperSaturationLimit=1  LowerSaturationLimit=0  LinearizeAsGain=on  AntiWindupMode=none  Kb=1  LimitIntegrator=off  UpperIntegratorSaturationLimit=inf  LowerIntegratorSaturationLimit=-inf  POutMin=[]  POutMax=[]  IOutMin=[]  IOutMax=[]  DOutMin=[]  DOutMax=[]  NOutMin=[]  NOutMax=[]  SumOutMin=[]  SumOutMax=[]  SaturationOutMin=[]  SaturationOutMax=[]  PParamMin=[]  PParamMax=[]  IParamMin=[]  IParamMax=[]  DParamMin=[]  DParamMax=[]  NParamMin=[]  NParamMax=[]  KbParamMin=[]  KbParamMax=[]  KtParamMin=[]  KtParamMax=[]  KbOutMin=[]  KbOutMax=[]  KtOutMin=[]  KtOutMax=[]  IntegratorOutMin=[]  IntegratorOutMax=[]  FilterOutMin=[]  FilterOutMax=[]  SumI1OutMin=[]  SumI1OutMax=[]  SumI2OutMin=[]  SumI2OutMax=[]  SumI3OutMin=[]  SumI3OutMax=[]  SumI4OutMin=[]  SumI4OutMax=[]  SumDOutMin=[]  SumDOutMax=[]  DifferentiatorOutMin=[]  DifferentiatorOutMax=[]  FilterDiffOutCoefMin=[]  FilterDiffOutCoefMax=[]  ReciprocalOutMin=[]  ReciprocalOutMax=[]  SumDenOutMin=[]  SumDenOutMax=[]  SumNumOutMin=[]  SumNumOutMax=[]  DivideOutMin=[]  DivideOutMax=[]  UdiffTsProdOutMin=[]  UdiffTsProdOutMax=[]  NTsProdOutMin=[]  NTsProdOutMax=[]  UintegralTsProdOutMin=[]  UintegralTsProdOutMax=[]  UngainTsProdOutMin=[]  UngainTsProdOutMax=[]  ClampingZeroOutDataTypeStr=Inherit: Inherit via back propagation  ClampingZeroOutMin=[]  ClampingZeroOutMax=[]  FilterDenConstantOutDataTypeStr=Inherit: Inherit via back propagation  FilterDenConstantOutMin=[]  FilterDenConstantOutMax=[]  PCopyOutDataTypeStr=Inherit: Inherit via back propagation  PCopyOutMin=[]  PCopyOutMax=[]  NCopyOutDataTypeStr=Inherit: Inherit via back propagation  NCopyOutMin=[]  NCopyOutMax=[]  IntegratorContinuousStateAttributes=''  IntegratorStateMustResolveToSignalObject=off  IntegratorRTWStateStorageClass=Auto  FilterContinuousStateAttributes=''  FilterStateMustResolveToSignalObject=off  FilterRTWStateStorageClass=Auto  ParallelPVariant=InternalParameters  IdealPVariant=Disabled  IVariant=InternalParameters  DVariant=Disabled  IntegratorVariant=Discrete  SatVariant=Enabled  AWVariant=Passthrough  PCopyVariant=Disabled  TRVariant=Disabled  FdbkBlocksVariant=Forward  IdealPFdbkVariant=Disabled  SatFdbkVariant=Disabled  DerivativeFilterVariant=Disabled  NVariant=Disabled  NCopyVariant=Disabled_SignalSpec  FilterICVariant=Disabled  IntegratorICVariant=InternalICs  ExternalResetVariant=Disabled  TRSumVariant=Passthrough  SumFdbkVariant=Disabled  SumVariant=Sum_PI  TsampFilterVariant=InternalTs  TsampNgainVariant=Passthrough  TsampIntegralVariant=Disabled_SignalSpec  ExternalSaturationOutDataTypeStr=Inherit: Same as second input  DerivativeSourceVariant=Disabled  PreIntVariant=InternalPreInt
  pu->SI : Gain  Gain=Vrms / sqrt(3) * sqrt(2)
  Vabc_inv : Outport
  ModWave : Outport  Port=2
  tag scope: V_1=global, freq_mea1=global
  wires:
  Vd Discrete PI Controller/1 -> Mux2/1  "Vd inverter"
  Mux2/1 -> Inverse Park Transform/1
  Sum1/1 -> Vd Discrete PI Controller/1
  Park Transform/1 -> Demux/1
  Sum2/1 -> Vq Discrete PI Controller/1
  Demux/2 -> Sum2/1
  Vq Discrete PI Controller/1 -> Mux2/2  "Vq inverter"
  V0/1 -> Mux2/3
  Demux/1 -> Sum1/2
  Demux/3 -> Terminator2/1
  "Sinusoidal Measurement (PLL, Three-Phase)"/3 -> [V_1]
  "Sinusoidal Measurement (PLL, Three-Phase)"/2 -> Inverse Park Transform/2, Park Transform/2
  "Sinusoidal Measurement (PLL, Three-Phase)"/1 -> [freq_mea1]
  Constant/1 -> "PWM Generator (Three-phase, Two-level)"/2
  Inverse Park Transform/1 -> pu->SI/1
  "PWM Generator (Three-phase, Two-level)"/1 -> Unit Delay1/1
  "PWM Generator (Three-phase, Two-level)"/2 -> Unit Delay2/1
  Unit Delay1/1 -> Vabc_inv/1
  pu->SI/1 -> "PWM Generator (Three-phase, Two-level)"/1
  Vabc (pu)/1 -> Power Measurement (Three-Phase)/1, Park Transform/1, "Sinusoidal Measurement (PLL, Three-Phase)"/1
  Iabc (pu)/1 -> Power Measurement (Three-Phase)/2
  Power Measurement (Three-Phase)/1 -> Sum3/2  "Inverter Active Power (pu)"
  Power Measurement (Three-Phase)/2 -> Sum/1  "nverter Reactive Power (pu)"
  P0/1 -> Sum3/1
  Q0/1 -> Sum/2
  Sum/1 -> Kqv/1
  Sum3/1 -> Kpf/1
  Kpf/1 -> Sum5/2
  Kqv/1 -> Sum4/1
  f0/1 -> Sum7/2
  Vref (pu)/1 -> Sum4/2
  Sum7/1 -> Sum5/1
  [freq_mea1] -> Sum7/1
  Sum5/1 -> Sum6/2
  Sum4/1 -> Sum8/2
  [freq_cmd] -> DQ Voltage Reference/1(freq_cmd)
  [V_cmd] -> DQ Voltage Reference/2(V_cmd)
  DQ Voltage Reference/1(Vd_ref) -> Sum1/1
  DQ Voltage Reference/2(Vq_ref) -> Sum2/2
  Unit Delay2/1 -> ModWave/1
  [freq_mea2] -> Transport Delay/1
  [freq_mea1] -> MATLAB Function/1(omega_1)
  Discrete-Time Integrator/1 -> MATLAB Function/6(int_v_in)
  Discrete-Time Integrator1/1 -> MATLAB Function/5(int_w_in)
  [V_1] -> MATLAB Function/3(V_1)
  Constant1/1 -> MATLAB Function/7(Ts)
  MATLAB Function/1(d_omega) -> Gain/1
  MATLAB Function/4(int_v_out) -> Discrete-Time Integrator/1
  MATLAB Function/3(int_w_out) -> Discrete-Time Integrator1/1
  Gain/1 -> Gain1/1
  Sum6/1 -> [freq_cmd]
  Sum8/1 -> [V_cmd]
  MATLAB Function/2(d_V) -> Gain2/1
  Transport Delay/1 -> MATLAB Function/2(omega_2)
  [V_2] -> Transport Delay1/1
  Transport Delay1/1 -> MATLAB Function/4(V_2)
  Gain1/1 -> Scope1/1, Sum6/1  "d_omega1"
  Gain2/1 -> Scope1/2, Sum8/1  "d_V1"
